simulink model "Ass2_extraB_PostureRegulation"  (R2024b)
settings: Solver=FixedStepAuto  StartTime=0.0  StopTime=inf  FixedStep=1/f_sim  RelTol=1e-3
values from neighbouring files (symbols this model uses):
  f_cmd = 100    [Main_ass2_extraB_PostureRegulation.m]
  f_odom = 100    [Main_ass2_extraB_PostureRegulation.m]
  K1 = 3    [Main_ass2_extraB_PostureRegulation.m]
  K2 = 3    [Main_ass2_extraB_PostureRegulation.m]
  K3 = 0.8    [Main_ass2_extraB_PostureRegulation.m]
  N = length(x_way)    [Main_ass2_extraB_PostureRegulation.m]
  r_slow = 0.4    [Main_ass2_extraB_PostureRegulation.m]
  toll_dist = 0.01    [Main_ass2_extraB_PostureRegulation.m]
  v_max = 0.5    [Main_ass2_extraB_PostureRegulation.m]
  v_min = -0.5    [Main_ass2_extraB_PostureRegulation.m]
  w_max = 2.84    [Main_ass2_extraB_PostureRegulation.m]
  w_min = -2.84    [Main_ass2_extraB_PostureRegulation.m]
  waypoints = [x_way' y_way' orient_way']    [Main_ass2_extraB_PostureRegulation.m]
undefined symbols (not defined in the file or in its folder): Angular, Linear
libraries: robotlib x3, simulink x3, hdlsllib x1
settings Model: Creator=vise  LastModifiedBy=vise
settings OptimizationCC: DefaultParameterBehavior=Inlined  EnhancedBackFolding=on  PassReuseOutputArgsAs=Individual arguments  ZeroExternalMemoryAtStartup=off  ZeroInternalMemoryAtStartup=off  MaxStackSize=64  OptimizeBlockOrder=speed  DifferentSizesBufferReuse=on  OptimizationCustomize=off  EfficientTunableParamExpr=on
settings DebuggingCC: ParameterTunabilityLossMsg=error
settings HardwareCC: ProdBitPerPointer=32  ProdBitPerSizeT=32  ProdBitPerPtrDiffT=32  ProdLargestAtomicFloat=None  ProdIntDivRoundTo=Undefined  ProdEndianess=Unspecified  ProdWordSize=32  ProdHWDeviceType=Generic->Unspecified (assume 32-bit Generic)  UseEmbeddedCoderFeatures=off
settings SFSimCC: MATLABDynamicMemAlloc=off
settings RTWCC: Description=Embedded Coder  SystemTargetFile=ert.tlc  HardwareBoard=Robot Operating System (ROS)  TLCOptions="-aInlineSetEventsForThisBaseRateFcn=TLC_FALSE -aSuppressMultiTaskScheduler=TLC_FALSE  -aRateBasedStepFcn=0"  TemplateMakefile=ert_default_tmf  Toolchain=Catkin  TargetLang=C++
settings CodeAppCC: ForceParamTrailComments=on  IgnoreCustomStorageClasses=off  OperatorAnnotations=on  SimulinkDataObjDesc=on  SFDataObjDesc=on  InsertBlockDesc=on
settings ERTTargetCC: SupportNonInlinedSFcns=on

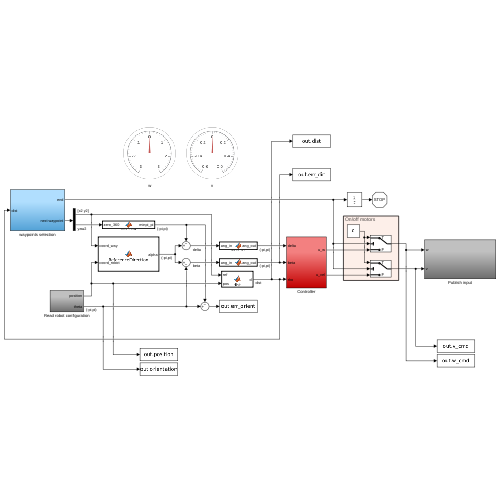
[thumbnail: Simulink's stored preview of the top-level diagram]
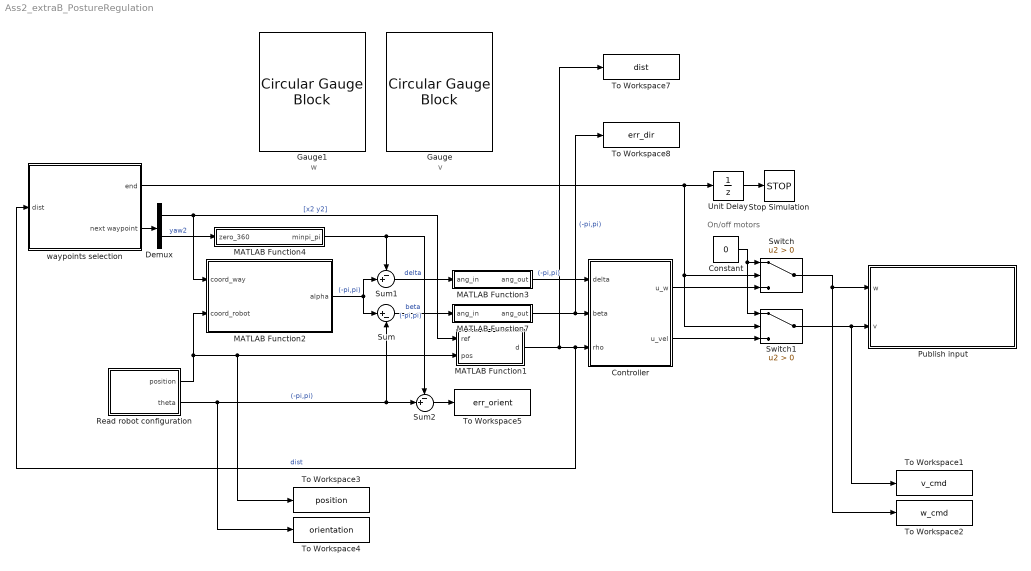
== system Ass2_extraB_PostureRegulation ==
  note: v
  note: On/off motors
  note: w
  Constant : Constant  Value=0
  Controller : Subsystem
  Demux : Demux  Outputs=2
  Gauge : CircularGaugeBlock  LabelPosition=Hide  ScaleMin=-0.6  ScaleMax=0.6
  Gauge1 : CircularGaugeBlock  LabelPosition=Hide  ScaleMin=-3  ScaleMax=3
  MATLAB Function1 : MATLAB Function  TreatAsAtomicUnit=on
  MATLAB Function2 : MATLAB Function  TreatAsAtomicUnit=on
  MATLAB Function3 : MATLAB Function  TreatAsAtomicUnit=on
  MATLAB Function4 : MATLAB Function  TreatAsAtomicUnit=on
  MATLAB Function7 : MATLAB Function  TreatAsAtomicUnit=on
  Publish input : Subsystem
  Read robot configuration : Subsystem
  Stop Simulation : Stop
  Sum : Sum  Inputs=|+-
  Sum1 : Sum  Inputs=-+|
  Sum2 : Sum  Inputs=-+|
  Switch : Switch  Criteria=u2 > Threshold  SaturateOnIntegerOverflow=off  InputSameDT=off
  Switch1 : Switch  Criteria=u2 > Threshold  SaturateOnIntegerOverflow=off  InputSameDT=off
  To Workspace1 : ToWorkspace  VariableName=v_cmd  SampleTime=-1
      settings: Save2DSignal=2-D array (concatenate along first dimension)
  To Workspace2 : ToWorkspace  VariableName=w_cmd  SampleTime=-1
      settings: Save2DSignal=2-D array (concatenate along first dimension)
  To Workspace3 : ToWorkspace  VariableName=position  SampleTime=-1
      settings: Save2DSignal=2-D array (concatenate along first dimension)
  To Workspace4 : ToWorkspace  VariableName=orientation  SampleTime=-1
      settings: Save2DSignal=2-D array (concatenate along first dimension)
  To Workspace5 : ToWorkspace  VariableName=err_orient  SampleTime=-1
      settings: Save2DSignal=2-D array (concatenate along first dimension)
  To Workspace7 : ToWorkspace  VariableName=dist  SampleTime=-1
      settings: Save2DSignal=2-D array (concatenate along first dimension)
  To Workspace8 : ToWorkspace  VariableName=err_dir  SampleTime=-1
      settings: Save2DSignal=2-D array (concatenate along first dimension)
  Unit Delay : UnitDelay  SampleTime=3  HasFrameUpgradeWarning=on
  waypoints selection : Subsystem
  wires:
  Demux/1 -> MATLAB Function2/1(coord_way), MATLAB Function1/1(ref)  "[x2 y2]"
  MATLAB Function1/1(d) -> waypoints selection/1(dist), Controller/3(rho), To Workspace7/1  "dist"
  MATLAB Function2/1(alpha) -> Sum/1, Sum1/2  "(-pi,pi)"
  Demux/2 -> MATLAB Function4/1(zero_360)  "yaw2"
  Sum/1 -> MATLAB Function7/1(ang_in)  "beta"
  Read robot configuration/2(theta) -> To Workspace4/1, Sum2/2, Sum/2  "(-pi,pi)"
  waypoints selection/2(next waypoint) -> Demux/1
  waypoints selection/1(end) -> Switch1/2, Switch/2, Unit Delay/1
  Switch/1 -> To Workspace2/1, Publish input/1(w)
  Switch1/1 -> To Workspace1/1, Publish input/2(v)
  Constant/1 -> Switch1/1, Switch/1
  Read robot configuration/1(position) -> MATLAB Function2/2(coord_robot), To Workspace3/1, MATLAB Function1/2(pos)
  Sum1/1 -> MATLAB Function3/1(ang_in)  "delta"
  Unit Delay/1 -> Stop Simulation/1
  MATLAB Function7/1(ang_out) -> To Workspace8/1, Controller/2(beta)  "(-pi,pi)"
  MATLAB Function4/1(minpi_pi) -> Sum2/1, Sum1/1  "(-pi,pi)"
  Controller/1(u_w) -> Switch/3
  Controller/2(u_vel) -> Switch1/3
  MATLAB Function3/1(ang_out) -> Controller/1(delta)  "(-pi,pi)"
  Sum2/1 -> To Workspace5/1

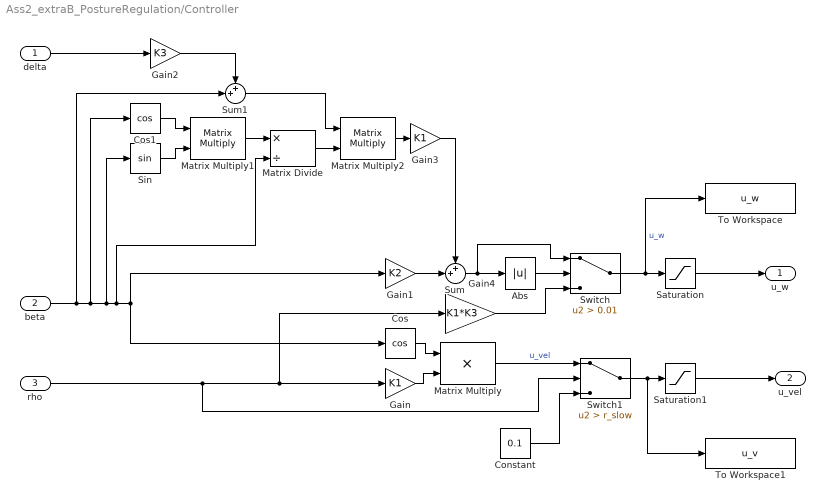
== system Ass2_extraB_PostureRegulation/Controller ==
  delta : Inport
  beta : Inport  Port=2
  rho : Inport  Port=3
  Abs : Abs  SaturateOnIntegerOverflow=off
  Constant : Constant  Value=0.1
  Cos : Trigonometry  Operator=cos
  Cos1 : Trigonometry  Operator=cos
  Gain : Gain  Gain=K1
  Gain1 : Gain  Gain=K2
  Gain2 : Gain  Gain=K3
  Gain3 : Gain  Gain=K1
  Gain4 : Gain  Gain=K1*K3
  Matrix Divide : Product  Inputs=*/
  Matrix Multiply : Product
  Matrix Multiply1 : Product  Multiplication=Matrix(*)
  Matrix Multiply2 : Product  Multiplication=Matrix(*)
  Saturation : Saturate  UpperLimit=w_max  LowerLimit=w_min
  Saturation1 : Saturate  UpperLimit=v_max  LowerLimit=v_min
  Sin : Trigonometry
  Sum : Sum  Inputs=++|
  Sum1 : Sum  Inputs=++|
  Switch : Switch  Criteria=u2 > Threshold  Threshold=0.01  SaturateOnIntegerOverflow=off  InputSameDT=off
  Switch1 : Switch  Criteria=u2 > Threshold  Threshold=r_slow  SaturateOnIntegerOverflow=off  InputSameDT=off
  To Workspace : ToWorkspace  VariableName=u_w  SampleTime=-1
      settings: Save2DSignal=2-D array (concatenate along first dimension)
  To Workspace1 : ToWorkspace  VariableName=u_v  SampleTime=-1
      settings: Save2DSignal=2-D array (concatenate along first dimension)
  u_w : Outport
  u_vel : Outport  Port=2
  wires:
  Gain4/1 -> Switch/3
  Switch/1 -> Saturation/1, To Workspace/1  "u_w"
  Sum/1 -> Abs/1, Switch/1
  Gain3/1 -> Sum/1
  Matrix Multiply2/1 -> Gain3/1
  Gain2/1 -> Sum1/1
  delta/1 -> Gain2/1
  Sum1/1 -> Matrix Multiply2/1
  Matrix Divide/1 -> Matrix Multiply2/2
  Matrix Multiply1/1 -> Matrix Divide/1
  Sin/1 -> Matrix Multiply1/2
  Cos1/1 -> Matrix Multiply1/1
  Gain1/1 -> Sum/2
  Gain/1 -> Matrix Multiply/2
  Cos/1 -> Matrix Multiply/1
  beta/1 -> Matrix Divide/2, Cos/1, Gain1/1, Sin/1, Cos1/1, Sum1/2
  rho/1 -> Switch1/2, Gain/1, Gain4/1
  Matrix Multiply/1 -> Switch1/1  "u_vel"
  Saturation1/1 -> u_vel/1
  Saturation/1 -> u_w/1
  Abs/1 -> Switch/2
  Switch1/1 -> To Workspace1/1, Saturation1/1
  Constant/1 -> Switch1/3

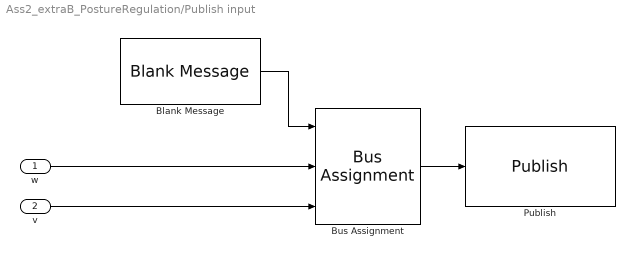
== system Ass2_extraB_PostureRegulation/Publish input ==
  w : Inport
  v : Inport  Port=2
  Blank Message : robotlib/Blank Message  messageClass=Message  entityType=geometry_msgs/Twist  messageType=geometry_msgs/Twist  SampleTime=1/f_cmd  legacyBusStruct=off
  Bus Assignment : BusAssignment  AssignedSignals=Angular.Z,Linear.X
  Publish : robotlib/Publish  topicSource=Select from ROS network  topic=/cmd_vel  messageType=geometry_msgs/Twist  legacyBusStruct=off  messageQueueLength=1
  wires:
  Bus Assignment/1 -> Publish/1
  Blank Message/1 -> Bus Assignment/1
  v/1 -> Bus Assignment/3
  w/1 -> Bus Assignment/2

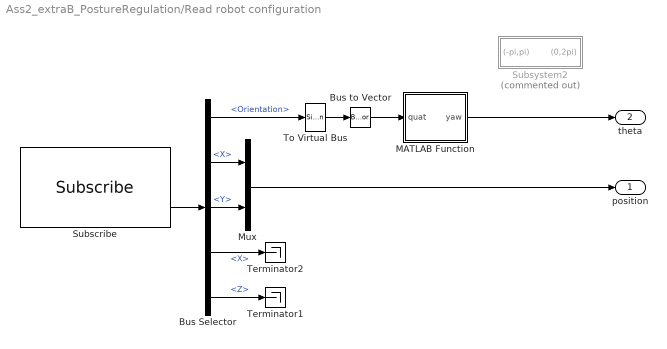
== system Ass2_extraB_PostureRegulation/Read robot configuration ==
  Bus Selector : BusSelector  OutputSignals=Pose.Pose.Orientation,Pose.Pose.Position.X,Pose.Pose.Position.Y,Twist.Twist.Linear.X,Twist.Twist.Angular.Z
  Bus to Vector : BusToVector
  MATLAB Function : MATLAB Function  TreatAsAtomicUnit=on
  Mux : Mux  Inputs=2
  Subscribe : robotlib/Subscribe  topicSource=Select from ROS network  topic=/odom  messageType=nav_msgs/Odometry  SampleTime=1/f_odom  legacyBusStruct=off  messageQueueLength=1
  Subsystem2 : Subsystem  Commented=on
  Terminator1 : Terminator
  Terminator2 : Terminator
  To Virtual Bus : SignalConversion  ConversionOutput=Virtual bus  OverrideOpt=off
  position : Outport
  theta : Outport  Port=2
  wires:
  Bus to Vector/1 -> MATLAB Function/1(quat)
  Mux/1 -> position/1
  Bus Selector/1 -> To Virtual Bus/1  "<Orientation>"
  Bus Selector/2 -> Mux/1  "<X>"
  To Virtual Bus/1 -> Bus to Vector/1
  Subscribe/2 -> Bus Selector/1
  Bus Selector/3 -> Mux/2  "<Y>"
  MATLAB Function/1(yaw) -> theta/1
  Bus Selector/4 -> Terminator2/1  "<X>"
  Bus Selector/5 -> Terminator1/1  "<Z>"

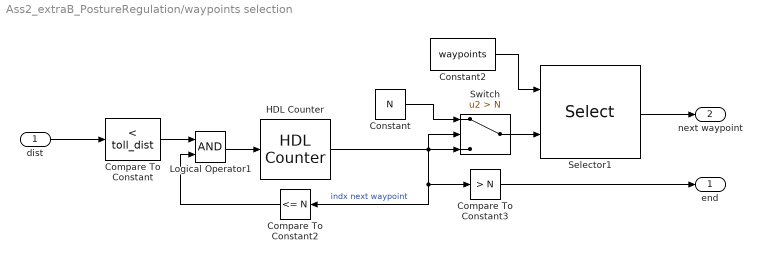
== system Ass2_extraB_PostureRegulation/waypoints selection ==
  dist : Inport
  Compare To Constant : simulink/Logic and Bit Operations/Compare To Constant  relop=<  const=toll_dist  OutDataTypeStr=boolean
  Compare To Constant2 : simulink/Logic and Bit Operations/Compare To Constant  relop=<=  const=N  OutDataTypeStr=boolean
  Compare To Constant3 : simulink/Logic and Bit Operations/Compare To Constant  relop=>  const=N  OutDataTypeStr=boolean
  Constant : Constant  Value=N
  Constant2 : Constant  Value=waypoints
  HDL Counter : hdlsllib/Sources/HDL Counter  CountType=Count limited  CountInit=1  CountStep=1  CountMax=N+1  CountFromType=Initial value  CountFrom=1  CountResetPort=off  CountLoadPort=off  CountEnbPort=on  CountDirPort=off  CountHitOutputPort=off  CountDataType=Unsigned  CountWordLen=8  CountFracLen=0  CountSampTime=1
  Logical Operator1 : Logic  AllPortsSameDT=off  OutDataTypeStr=boolean
  Selector1 : Selector  NumberOfDimensions=2  InputPortWidth=3  IndexOptions=Index vector (port),Select all  Indices=[1 3],[1 2]  OutputSizes=1,1
  Switch : Switch  Criteria=u2 > Threshold  Threshold=N  SaturateOnIntegerOverflow=off  InputSameDT=off
  end : Outport
  next waypoint : Outport  Port=2
  wires:
  HDL Counter/1 -> Compare To Constant3/1, Compare To Constant2/1, Switch/3, Switch/2  "indx next waypoint"
  Compare To Constant/1 -> Logical Operator1/1
  dist/1 -> Compare To Constant/1
  Selector1/1 -> next waypoint/1
  Constant2/1 -> Selector1/1
  Logical Operator1/1 -> HDL Counter/1
  Compare To Constant2/1 -> Logical Operator1/2
  Switch/1 -> Selector1/2
  Constant/1 -> Switch/1
  Compare To Constant3/1 -> end/1

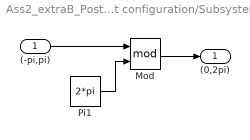
== system Ass2_extraB_PostureRegulation/Read robot configuration/Subsystem2 ==
  (-pi,pi) : Inport
  Mod : Math  Operator=mod
  Pi1 : Constant  Value=2*pi  OutDataTypeStr=Inherit: Inherit via back propagation
  (0,2pi) : Outport
  wires:
  Mod/1 -> (0,2pi)/1
  Pi1/1 -> Mod/2
  (-pi,pi)/1 -> Mod/1

== matlab function Ass2_extraB_PostureRegulation/Read robot configuration/MATLAB Function ==
  data: quat input; yaw output
function yaw=quat2yaw(quat)

q=zeros(1,4);

q(1)=quat(1);
q(2)=quat(2);
q(3)=quat(3);
q(4)=quat(4);

eul=quat2eul(q);

yaw=eul(3);

end

== matlab function Ass2_extraB_PostureRegulation/MATLAB Function2 ==
  data: coord_way input; alpha output; coord_robot input
function alpha=ReferenceDirection(coord_way,coord_robot)

% computes the direction (angle wrt positive x axis,
% counterclockwise) between two inputed points [x1 y1 ; x2 y2] 

x1=coord_robot(1);
y1=coord_robot(2);
x2=coord_way(1);
y2=coord_way(2);

alpha=atan2((y2-y1),(x2-x1)); % (-pi,pi)

%alpha=mod(alpha,2*pi); % (0,2pi)

end

== matlab function Ass2_extraB_PostureRegulation/MATLAB Function4 ==
  data: zero_360 input; minpi_pi output
function minpi_pi=convert(zero_360)

if zero_360<pi
    minpi_pi=zero_360;
else
    minpi_pi=zero_360-2*pi;
end

end

== matlab function Ass2_extraB_PostureRegulation/MATLAB Function3 ==
  data: ang_in input; ang_out output
function ang_out=mpi_pi(ang_in)

% Impose angle to be within (-pi,pi)

if ang_in<=pi && ang_in>=-pi
    ang_out=ang_in;
else
    ang_out=mod(ang_in+pi, 2*pi)-pi;
end

end

== matlab function Ass2_extraB_PostureRegulation/MATLAB Function7 ==
  data: ang_in input; ang_out output
function ang_out=mpi_pi(ang_in)

% Impose angle to be within (-pi,pi)

if ang_in<=pi && ang_in>=-pi
    ang_out=ang_in;
else
    ang_out=mod(ang_in+pi, 2*pi)-pi;
end

end

== matlab function Ass2_extraB_PostureRegulation/MATLAB Function1 ==
  data: ref input; d output; pos input
function d=dist(ref,pos)

% computes the distance between two points (x1,y1) and (x2,y2)

x_ref=ref(1);
y_ref=ref(2);
x_pos=pos(1);
y_pos=pos(2);

d=sqrt((x_ref-x_pos)^2+(y_ref-y_pos)^2);

end
